simulink model "DT_EOPLL"  (R2023b)
settings: Solver=VariableStepAuto  StartTime=0.0  StopTime=1e-1  RelTol=1e-11
values from neighbouring files (symbols this model uses):
  f0 = 5e9    (= 5000000000)    [CT_EOPLL.m]    (also in DT_EOPLL.m = 50000000000)
  h0 = 1e4    (= 10000)    [CT_EOPLL.m]    (also in DT_EOPLL.m)
  K_int = 10    [CT_EOPLL.m]    (also in DT_EOPLL.m)
  K_loop = 3.33e-3    (= 0.00333)    [CT_EOPLL.m]    (also in DT_EOPLL.m = 10)
  Kf = 1e13    (= 10000000000000)    [CT_EOPLL.m]    (also in DT_EOPLL.m)
  p0 = 1    [CT_EOPLL.m]    (also in DT_EOPLL.m)
  R = 1    [CT_EOPLL.m]    (also in DT_EOPLL.m)
  T_meas = 2e-4    (= 0.0002)    [CT_EOPLL.m]    (also in DT_EOPLL.m)
  t_mzi = 2e-9    (= 2e-09)    [CT_EOPLL.m]    (also in DT_EOPLL.m = 2e-08)
  t_pfd = 1e-9    (= 1e-09)    [DT_EOPLL.m]
  T_ref = 5e-7    (= 5e-07)    [DT_EOPLL.m]
  w_int = 2*pi*300    (= 1884.95559215)    [CT_EOPLL.m]    (also in DT_EOPLL.m)
  wf = 2*pi*1e7    (= 62831853.0718)    [CT_EOPLL.m]    (also in DT_EOPLL.m)
  wz = 2*pi*100.4e3    (= 630831.804841)    [DT_EOPLL.m]    (also in LoopPar_func_DTEOPLL.m = wz1(1))
undefined symbols (not defined in the file or in its folder): j, magnitude
libraries: simulink_extras x2, msbPllFoundation x1, simulink x1
settings Model: Creator=Marziyeh Rezaei  LastModifiedBy=Marziyeh Rezaei
settings DebuggingCC: UnconnectedInputMsg=warning  UnconnectedOutputMsg=warning  UnconnectedLineMsg=warning
settings ModelReferenceCC: EnableRefExpFcnMdlSchedulingChecks=on
settings RTWCC: DLArmComputeVersion=19.05

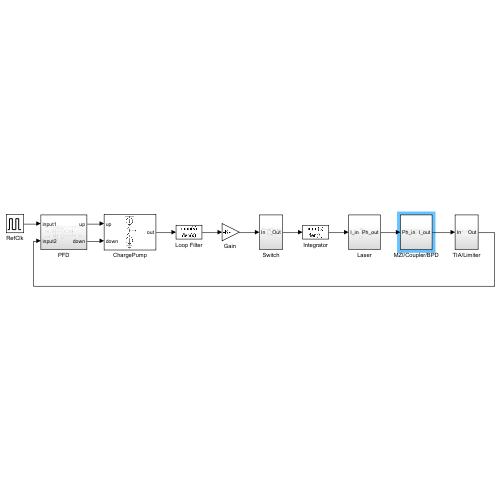
[thumbnail: Simulink's stored preview of the top-level diagram]
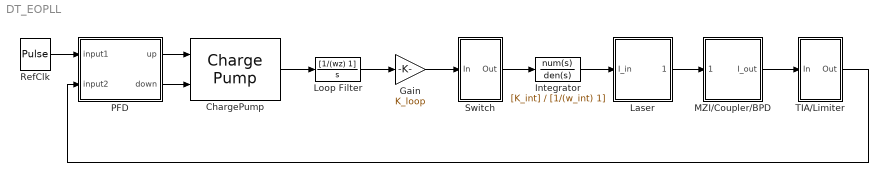
== system DT_EOPLL ==
  ChargePump : msbPllFoundation/Charge Pump  OutputCurrent=i_out  InputThreshold=vth  ExtraBuffer=off  NBuffer=10  EnableCurrentImpairments=off  CurrentImbalance=1e-7  LeakageCurrent=1e-8  EnableTimingImpairments=off  DefaultOrAdvanced=Default  MaxFreqInterest=10e9  RiseFallUp=5e-9  PropDelayUp=6e-9  RiseFallDown=2e-9  PropDelayDown=4e-9
  "Gain " : Gain  Gain=K_loop
  Integrator : TransferFcn  Numerator=[K_int]  Denominator=[1/(w_int) 1]
  Laser : Subsystem
  Loop Filter : TransferFcn  Numerator=[1/(wz) 1]  Denominator=[1 0]
  MZI/Coupler/BPD : Subsystem
  PFD : Subsystem
  RefClk : DiscretePulseGenerator  PulseType=Time based  Period=T_ref  PulseWidth=50  PhaseDelay=5e-5
  Switch : Subsystem
  TIA/Limiter : Subsystem
  wires:
  PFD/1(up) -> ChargePump/1
  RefClk/1 -> PFD/1(input1)
  PFD/2(down) -> ChargePump/2
  ChargePump/1 -> Loop Filter/1
  Loop Filter/1 -> "Gain "/1
  "Gain "/1 -> Switch/1(In)
  Switch/1(Out) -> Integrator/1
  TIA/Limiter/1(Out) -> PFD/2(input2)
  Integrator/1 -> Laser/1(I_in)
  Laser/1(Ph_out) -> MZI/Coupler/BPD/1(Ph_in)
  MZI/Coupler/BPD/1(I_out) -> TIA/Limiter/1(In)

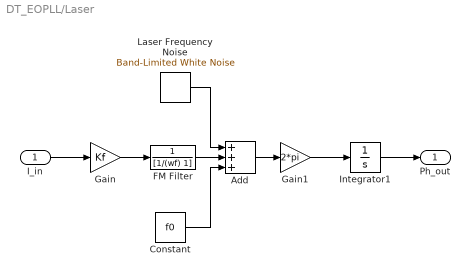
== system DT_EOPLL/Laser ==
  I_in : Inport
  Add : Sum  Inputs=+++
  Constant : Constant  Value=f0
  FM Filter : TransferFcn  Denominator=[1/(wf) 1]
  Gain : Gain  Gain=Kf
  Gain1 : Gain  Gain=2*pi
  Integrator1 : Integrator
  Laser Frequency Noise : simulink/Sources/Band-Limited White Noise  Cov=[h0]  Ts=2e-7  seed=[23341]
  Ph_out : Outport
  wires:
  Gain/1 -> FM Filter/1
  Gain1/1 -> Integrator1/1
  I_in/1 -> Gain/1
  Integrator1/1 -> Ph_out/1
  FM Filter/1 -> Add/2
  Add/1 -> Gain1/1
  Laser Frequency Noise/1 -> Add/1
  Constant/1 -> Add/3

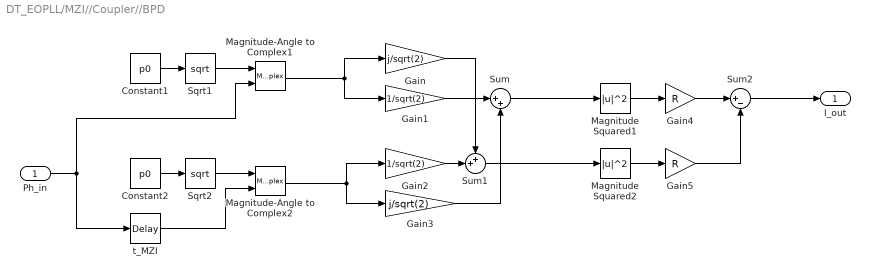
== system DT_EOPLL/MZI//Coupler//BPD ==
  Ph_in : Inport
  Constant1 : Constant  Value=p0
  Constant2 : Constant  Value=p0
  Gain : Gain  Gain=j/sqrt(2)
  Gain1 : Gain  Gain=1/sqrt(2)
  Gain2 : Gain  Gain=1/sqrt(2)
  Gain3 : Gain  Gain=j/sqrt(2)
  Gain4 : Gain  Gain=R
  Gain5 : Gain  Gain=R
  Magnitude Squared1 : Math  Operator=magnitude^2
  Magnitude Squared2 : Math  Operator=magnitude^2
  Magnitude-Angle to Complex1 : MagnitudeAngleToComplex
  Magnitude-Angle to Complex2 : MagnitudeAngleToComplex
  Sqrt1 : Sqrt
  Sqrt2 : Sqrt
  Sum : Sum  Inputs=|++
  Sum1 : Sum  Inputs=++|
  Sum2 : Sum  Inputs=|+-
  t_MZI : TransportDelay  DelayTime=t_mzi
  I_out : Outport
  wires:
  t_MZI/1 -> Magnitude-Angle to Complex2/2
  Sqrt1/1 -> Magnitude-Angle to Complex1/1
  Constant2/1 -> Sqrt2/1
  Ph_in/1 -> Magnitude-Angle to Complex1/2, t_MZI/1
  Sqrt2/1 -> Magnitude-Angle to Complex2/1
  Constant1/1 -> Sqrt1/1
  Gain4/1 -> Sum2/1
  Magnitude Squared2/1 -> Gain5/1
  Sum2/1 -> I_out/1
  Magnitude Squared1/1 -> Gain4/1
  Gain5/1 -> Sum2/2
  Gain3/1 -> Sum/2
  Magnitude-Angle to Complex1/1 -> Gain1/1, Gain/1
  Gain/1 -> Sum1/1
  Magnitude-Angle to Complex2/1 -> Gain2/1, Gain3/1
  Gain2/1 -> Sum1/2
  Gain1/1 -> Sum/1
  Sum/1 -> Magnitude Squared1/1
  Sum1/1 -> Magnitude Squared2/1

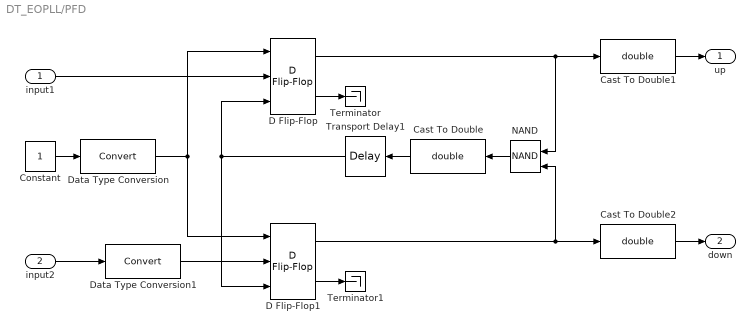
== system DT_EOPLL/PFD ==
  input1 : Inport
  input2 : Inport  Port=2
  Cast To Double : DataTypeConversion  OutDataTypeStr=double  SaturateOnIntegerOverflow=off  RndMeth=Floor
  Cast To Double1 : DataTypeConversion  OutDataTypeStr=double  SaturateOnIntegerOverflow=off  RndMeth=Floor
  Cast To Double2 : DataTypeConversion  OutDataTypeStr=double  SaturateOnIntegerOverflow=off  RndMeth=Floor
  Constant : Constant
  D Flip-Flop : simulink_extras/Flip Flops/D Flip-Flop
  D Flip-Flop1 : simulink_extras/Flip Flops/D Flip-Flop
  Data Type Conversion : DataTypeConversion  SaturateOnIntegerOverflow=off  RndMeth=Floor
  Data Type Conversion1 : DataTypeConversion  SaturateOnIntegerOverflow=off  RndMeth=Floor
  NAND : Logic  Operator=NAND  IconShape=distinctive  AllPortsSameDT=off  OutDataTypeStr=boolean
  Terminator : Terminator
  Terminator1 : Terminator
  Transport Delay1 : TransportDelay  DelayTime=t_pfd
  up : Outport
  down : Outport  Port=2
  wires:
  D Flip-Flop/1 -> Cast To Double1/1, NAND/1
  Constant/1 -> Data Type Conversion/1
  D Flip-Flop1/1 -> Cast To Double2/1, NAND/2
  Cast To Double/1 -> Transport Delay1/1
  D Flip-Flop/2 -> Terminator/1
  Data Type Conversion/1 -> D Flip-Flop1/1, D Flip-Flop/1
  NAND/1 -> Cast To Double/1
  Transport Delay1/1 -> D Flip-Flop1/3, D Flip-Flop/3
  input2/1 -> Data Type Conversion1/1
  input1/1 -> D Flip-Flop/2
  D Flip-Flop1/2 -> Terminator1/1
  Cast To Double1/1 -> up/1
  Cast To Double2/1 -> down/1
  Data Type Conversion1/1 -> D Flip-Flop1/2

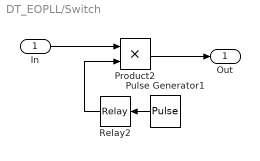
== system DT_EOPLL/Switch ==
  In : Inport
  Product2 : Product
  Pulse Generator1 : DiscretePulseGenerator  PulseType=Time based  Period=T_meas  PulseWidth=50  PhaseDelay=1e-4
  Relay2 : Relay  OnSwitchValue=1  OffSwitchValue=0  OffOutputValue=-1
  Out : Outport
  wires:
  Relay2/1 -> Product2/2
  Pulse Generator1/1 -> Relay2/1
  Product2/1 -> Out/1
  In/1 -> Product2/1

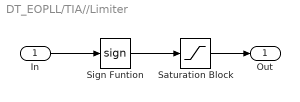
== system DT_EOPLL/TIA//Limiter ==
  In : Inport
  Saturation Block : Saturate  UpperLimit=1  LowerLimit=0
  Sign Funtion : Signum
  Out : Outport
  wires:
  Sign Funtion/1 -> Saturation Block/1
  In/1 -> Sign Funtion/1
  Saturation Block/1 -> Out/1
